simulink model "Week13_Sim4"  (R2021a)
settings: Solver=VariableStepAuto  StartTime=0.0  StopTime=10.0  RelTol=1e-3
values from neighbouring files (symbols this model uses):
  C = 10e-6    (= 1e-05)    [Week13_Ex1.m]    (also in Week13_Ex2.m = 0.0001; Week13_Ex3.m = 0.0001; Week13_Ex4.m = 0.0001)
  L = 2.5    [Week13_Ex1.m]    (also in Week13_Ex2.m; Week13_Ex3.m; Week13_Ex4.m)
  R = 100    [Week13_Ex1.m]    (also in Week13_Ex2.m; Week13_Ex3.m; Week13_Ex4.m)
  ws = 20    [Week13_Ex4.m]
settings Model: Creator=wesmcevoy  LastModifiedBy=wesmcevoy

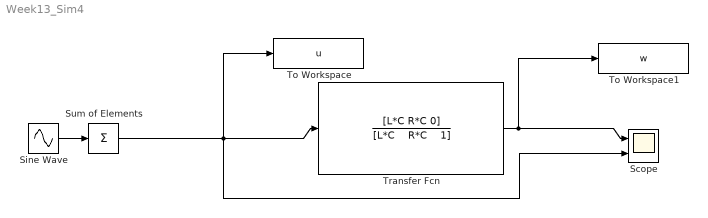
== system Week13_Sim4 ==
  Scope : Scope  NumInputPorts=2
  Sine Wave : Sin  Frequency=ws  Phase=2*pi*rand(1,200)  SampleTime=0
  Sum of Elements : Sum  Inputs=+
  To Workspace : ToWorkspace  VariableName=u  SampleTime=-1
  To Workspace1 : ToWorkspace  VariableName=w  SampleTime=-1
  Transfer Fcn : TransferFcn  Numerator=[L*C R*C 0]  Denominator="[L*C    R*C    1]"
  wires:
  Transfer Fcn/1 -> Scope/1, To Workspace1/1
  Sine Wave/1 -> Sum of Elements/1
  Sum of Elements/1 -> To Workspace/1, Transfer Fcn/1, Scope/2
